simulink model "Control_v6_LQR_2020b"  (R2020b)
settings: Solver=FixedStepAuto  StartTime=0.0  StopTime=t_sim  FixedStep=TimeStep  RelTol=1e-3
values from neighbouring files (symbols this model uses):
  R = [ 1    0            0;         0    cos(alpha)  -sin(alpha);         0    sin(alpha)   cos(alpha)]    [main_SCA_v3.m]    (also in main_SCA_v3_alt.m; main_SCA_v4_LQR.m; main_SCA_v5.m)
  Use_IGRF = 0    [main_SCA.m]    (also in main_SCA_v3.m; main_SCA_v3_alt.m; main_SCA_v4_LQR.m; main_SCA_v5.m = 1)
undefined symbols (not defined in the file or in its folder): att, C, date, deg, DiscIntNeverNeededParam, IonSataero, Isat_inverse, km, orbit, Q, rad, s, sat
libraries: vrlib x23, aerolibutil x16, dspmathops x15, aerolibconvert2 x14, sharedtransform x13, simulink x4, simulink_extras x2, aerolibatmos2 x1, DipoleModel x1, aerolibobsolete x1, sharedutil x1, aerolibcelestial x1
(part 2 of 4)

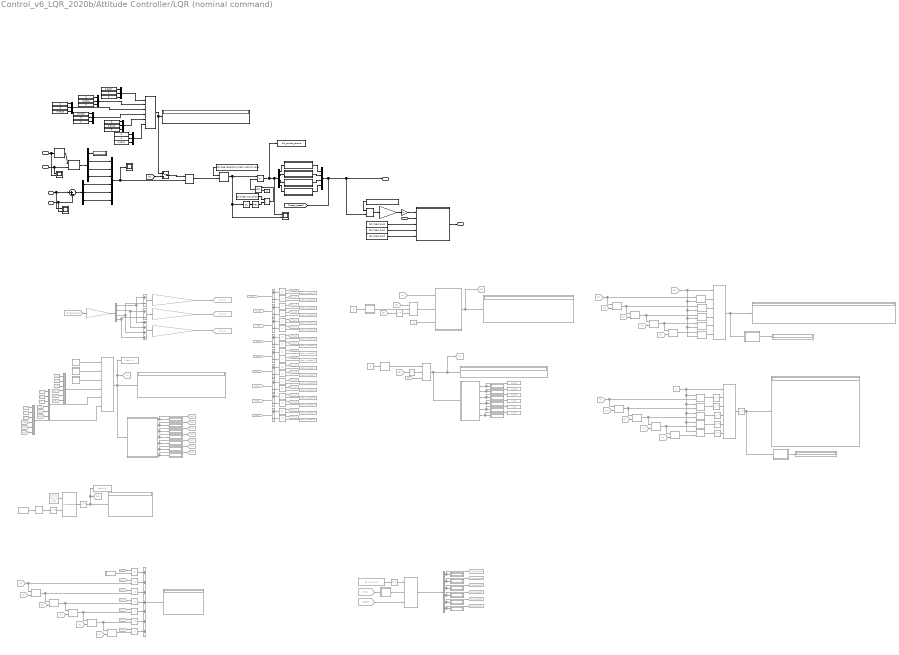
== system Control_v6_LQR_2020b/Attitude Controller/LQR (nominal command) ==
  note: Observability matrix [Ob]
  note: Feedback gain obtained by solving the algebraic Riccati equation
  note: Algebraic Riccati equation solver
  note: Feedback gain matrix K from the Ackerman's formula
  note: The dynamic of the corrected system is contained is the polynomial P_BF(A)
  note: State-space A matrix and its characteristic polynomial coefficients
  note: State-space B matrix
  note: Governability or Controllability matrix Gv
  note: on projete T dans
      | le plan perpendiculaire à B ?
      | Pas obligatoire (cf définition des blocs)
  note: See https://en.wikipedia.org/wiki/Rotation_formalisms_in_three_dimensions Quaternion <=> Angular velocity
      |
      | See http://www.diva-portal.org/smash/get/diva2:1020537/FULLTEXT02.pdf for 6DOF equations (3.13 p15)
      |
      | With ω = rotation vector (Omega_body) we have :
      |
      | $\frac{dω}{dt} = \hat{I}^{-1} [−ω(t) × (I_{Total}ω(t) + h_{RW}) + T_{dist}(t) − \frac{dh_{RW}}{dt} ̇ ]$
      | and with $\hat{I}=I_{Total}-L*I_{RW}*L^T$
  note: Computing the coefficient of the matrix A
  B_IGRF_Body : Inport
  q_ref : Inport  Port=2
  Q_ECI : Inport  Port=3
  W_Body : Inport  Port=4
  W_ref : Inport  Port=5
  Abs2 : Abs
  Algebraic Riccati equation solver : MATLAB Function  Commented=on  TreatAsAtomicUnit=on
  Command Magnetic moments computation : Subsystem
  Constant : Constant  Value=sat.wheel.repartition_matrix_4RW
  Constant1 : Constant  Commented=on  Value=[0 0 0 0 0 1]
  Constant10 : Constant  Commented=on  Value=Isat_inverse(7)
  Constant11 : Constant  Commented=on  Value=Isat_inverse(8)
  Constant12 : Constant  Value=sat.mag_t.axe1
  Constant13 : Constant  Value=sat.mag_t.axe2
  Constant14 : Constant  Value=sat.mag_t.axe3
  Constant15 : Constant  Commented=on  Value=Isat_inverse(9)
  Constant16 : Constant  Commented=on  Value=Isat_inverse(7)
  Constant17 : Constant  Commented=on  Value=Isat_inverse(8)
  Constant18 : Constant  Commented=on  Value=Isat_inverse(9)
  Constant19 : Constant  Commented=on  Value=Isat_inverse(1)
  Constant2 : Constant  Commented=on  Value=Isat_inverse(1)
  Constant20 : Constant  Commented=on  Value=Isat_inverse(2)
  Constant21 : Constant  Commented=on  Value=Isat_inverse(3)
  Constant22 : Constant  Commented=on  Value=Isat_inverse(4)
  Constant23 : Constant  Commented=on  Value=Isat_inverse(5)
  Constant24 : Constant  Commented=on  Value=Isat_inverse(6)
  Constant25 : Constant  Commented=on  Value=1/2
  Constant{26..28,30..32} (6 alike) : Constant  Commented=on  Value=0
  Constant29 : Constant  Commented=on  Value=1/2
  Constant3 : Constant  Commented=on  Value=Isat_inverse(2)
  Constant33 : Constant  Commented=on  Value=1/2
  Constant34 : Constant  Commented=on  Value=[0 0 0; 0 0 0; 0 0 0]
  Constant35 : Constant  Commented=on  Value=sat.inertia
  Constant36 : Constant  Commented=on  Value=R
  Constant37 : Constant  Value=sat.wheel.max_torque
  Constant38 : Constant
  Constant39 : Constant  Commented=on  Value=Q
  Constant4 : Constant  Commented=on  Value=Isat_inverse(3)
  Constant{6,40,42..43,46..48,51,53..56} (12 alike) : Constant  Value=0
  Constant41 : Constant  Commented=on  Value=R
  Constant44 : Constant  Value=0.0151
  Constant45 : Constant  Value=0.0017
  Constant49 : Constant  Value=0.0122
  Constant5 : Constant  Commented=on  Value=Isat_inverse(4)
  Constant50 : Constant  Commented=on  Value=C
  Constant52 : Constant  Value=0.0103
  Constant57 : Constant  Value=0.0016
  Constant7 : Constant  Value=0.0016
  Constant8 : Constant  Commented=on  Value=Isat_inverse(5)
  Constant9 : Constant  Commented=on  Value=Isat_inverse(6)
  Demux : Demux
  Demux4 : Demux  Commented=on
  Demux6 : Demux  Commented=on  Outputs=6
  Demux7 : Demux
  Demux8 : Demux  Outputs=3
  Display : Display
  Display{1..19,21..22,26,31..36} (28 alike) : Display  Commented=on
  Display20 : Display
  Divide1 : Product  Inputs=*/
  From : From  Commented=on  GotoTag=A44
  From100 : From  Commented=on  GotoTag=a6
  From{76..80,82..87,103,106,109..112} (17 alike) : From  Commented=on
  From{70,104..105,108} (4 alike) : From  Commented=on  GotoTag=B
  From107 : From  Commented=on  GotoTag=P
  From13 : From  Commented=on  GotoTag=Wheel_speed
  From31 : From  Commented=on  GotoTag=A54
  From32 : From  Commented=on  GotoTag=A64
  From33 : From  Commented=on  GotoTag=A45
  From{34,40,43,46,50,53} (6 alike) : From  Commented=on  GotoTag=hw_x
  From{35,41,44,47,56..57} (6 alike) : From  Commented=on  GotoTag=hw_z
  From{36,42,45,51..52,54} (6 alike) : From  Commented=on  GotoTag=hw_y
  From64 : From  Commented=on  GotoTag=A55
  From65 : From  Commented=on  GotoTag=A65
  From66 : From  Commented=on  GotoTag=A46
  From67 : From  Commented=on  GotoTag=A56
  From68 : From  Commented=on  GotoTag=A66
  From88 : From  Commented=on  GotoTag=Gv
  From89 : From  Commented=on  GotoTag=P_BF
  From94 : From  Commented=on  GotoTag=a0
  From95 : From  Commented=on  GotoTag=a1
  From96 : From  Commented=on  GotoTag=a2
  From97 : From  Commented=on  GotoTag=a3
  From98 : From  Commented=on  GotoTag=a4
  From99 : From  Commented=on  GotoTag=a5
  Gain1 : Gain
  Gain2 : Gain  Commented=on  Gain=sat.wheel.inertia
  Goto1 : Goto  Commented=on  GotoTag=A44
  Goto10 : Goto  Commented=on  GotoTag=A54
  Goto11 : Goto  Commented=on  GotoTag=hw_x
  Goto12 : Goto  Commented=on  GotoTag=hw_y
  Goto13 : Goto  Commented=on  GotoTag=hw_z
  Goto14 : Goto  Commented=on  GotoTag=A55
  Goto15 : Goto  Commented=on  GotoTag=A56
  Goto16 : Goto  Commented=on  GotoTag=A64
  Goto17 : Goto  Commented=on  GotoTag=A65
  Goto18 : Goto  Commented=on  GotoTag=A66
  Goto19 : Goto  Commented=on
  Goto2 : Goto  Commented=on  GotoTag=K
  Goto20 : Goto  Commented=on  GotoTag=B
  Goto21 : Goto  Commented=on  GotoTag=a5
  Goto23 : Goto  Commented=on  GotoTag=a4
  Goto24 : Goto  Commented=on  GotoTag=a3
  Goto25 : Goto  Commented=on  GotoTag=a2
  Goto26 : Goto  Commented=on  GotoTag=a1
  Goto27 : Goto  Commented=on  GotoTag=a0
  Goto28 : Goto  Commented=on  GotoTag=a6
  Goto30 : Goto  Commented=on  GotoTag=P
  Goto31 : Goto  Commented=on  GotoTag=k_que2_ack
  Goto32 : Goto  Commented=on  GotoTag=k_que3_ack
  Goto34 : Goto  Commented=on  GotoTag=k_wb1_ack
  Goto35 : Goto  Commented=on  GotoTag=k_wb2_ack
  Goto36 : Goto  Commented=on  GotoTag=k_wb3_ack
  Goto37 : Goto  Commented=on  GotoTag=k_que1_ack
  Goto8 : Goto  Commented=on  GotoTag=A45
  Goto9 : Goto  Commented=on  GotoTag=A46
  IdentityMatrix [6x6] : Subsystem  Description=Replaced Block  Commented=on  mask(Replaced Block){}
      mask help: This block has been replaced with an empty subsystem because it used functionality that is unavailable in Simulink R2020b.
      mask Display: fprintf('Replaced: %s\n','IdentityMatrix')
  Inverse nxn matrix : MATLAB Function  Commented=on  TreatAsAtomicUnit=on
  Inverse nxn matrix1 : MATLAB Function  Commented=on  TreatAsAtomicUnit=on
  Inverse nxn matrix2 : MATLAB Function  Commented=on  TreatAsAtomicUnit=on
  Invert 3x3 Matrix : aerolibutil/Invert  3x3 Matrix  Commented=on
  Is the system controllable? : MATLAB Function  Commented=on  TreatAsAtomicUnit=on
  Is the system observable? : MATLAB Function  Commented=on  TreatAsAtomicUnit=on
  Manual Switch : ManualSwitch
  Matrix Concatenate : Concatenate  Commented=on  NumInputs=6  Mode=Multidimensional array  ConcatenateDimension=2
  Matrix Concatenate1 : Concatenate  Commented=on  Mode=Multidimensional array  ConcatenateDimension=2
  Matrix Concatenate2 : Concatenate  Commented=on  NumInputs=6  Mode=Multidimensional array  ConcatenateDimension=2
  Matrix Concatenate3 : Concatenate  Commented=on  NumInputs=6  Mode=Multidimensional array  ConcatenateDimension=2
  Matrix Concatenate4 : Concatenate  NumInputs=6  Mode=Multidimensional array  ConcatenateDimension=2
  Matrix Multiply{,1..13,17..25} (23 alike) : Product  Commented=on  Multiplication=Matrix(*)
  Matrix Multiply14 : Product  Commented=on  Inputs=3  Multiplication=Matrix(*)
  Matrix Multiply15 : Product  Commented=on  Inputs=3  Multiplication=Matrix(*)
  Matrix Multiply16 : Product  Commented=on  Inputs=3  Multiplication=Matrix(*)
  MatrixMultiply1 : Product  Multiplication=Matrix(*)
  MatrixMultiply2 : Product  Multiplication=Matrix(*)
  MatrixMultiply3 : Product  Multiplication=Matrix(*)
  Max of Elements2 : MinMax  Function=max
  Min1 : MinMax  Inputs=2
  Mux : Mux
  Mux5 : Mux  Inputs=6
  Product{2..12,31..37,54..60} (25 alike) : Product  Commented=on
  Product13 : Product
  Quaternion Inverse : aerolibutil/Quaternion Inverse
  Quaternion Multiplication : aerolibutil/Quaternion Multiplication
  RW1 : Subsystem
  RW2 : Subsystem
  RW3 : Subsystem
  "RW4 " : Subsystem
  Repartition RWA1 : Constant  Value=sat.wheel.repartition_metrix_4RW_inverse
  Scope : Scope
  Scope1 : Scope  NumInputPorts=2
  Scope2 : Scope  NumInputPorts=2
  Scope3 : Scope  NumInputPorts=2
  Sum{7,11,13..21} (11 alike) : Sum  Commented=on  Inputs=+-
  Sum12 : Sum  Commented=on  Inputs=++++
  Sum25 : Sum  Inputs=|+-
  Sum26 : Sum  Commented=on  Inputs=+++++++
  To Workspace11 : ToWorkspace  VariableName=RW_control_torque  SaveFormat=Timeseries  SampleTime=-1
  To Workspace2 : ToWorkspace  Commented=on  VariableName=Matrix_A  SaveFormat=Timeseries  SampleTime=-1
  To Workspace3 : ToWorkspace  Commented=on  VariableName=Matrix_B  SaveFormat=Timeseries  SampleTime=-1
  To Workspace4 : ToWorkspace  Commented=on  VariableName=k_qe1  SaveFormat=Timeseries  SampleTime=-1
  To Workspace5 : ToWorkspace  Commented=on  VariableName=k_qe2  SaveFormat=Timeseries  SampleTime=-1
  To Workspace6 : ToWorkspace  Commented=on  VariableName=k_qe3  SaveFormat=Timeseries  SampleTime=-1
  To Workspace7 : ToWorkspace  Commented=on  VariableName=k_w1  SaveFormat=Timeseries  SampleTime=-1
  To Workspace8 : ToWorkspace  Commented=on  VariableName=k_w2  SaveFormat=Timeseries  SampleTime=-1
  To Workspace9 : ToWorkspace  Commented=on  VariableName=k_w3  SaveFormat=Timeseries  SampleTime=-1
  Transpose{,1..10} (11 alike) : Math  Commented=on  Operator=transpose  SaturateOnIntegerOverflow=on
  Vector Concatenate : Concatenate  Commented=on  NumInputs=6
  Vector Concatenate1 : Concatenate  Commented=on  NumInputs=6
  Vector Concatenate2 : Concatenate  Commented=on  NumInputs=6
  Vector Concatenate{3..8} (6 alike) : Concatenate  NumInputs=3
  "[0 ... 0]^T" : Subsystem  Commented=on
  "[0 .... 0]^T" : Subsystem  Commented=on
  "[0 0 0 0 0 0]^T " : Subsystem  Commented=on
  cos(beta) : Gain  Commented=on  Gain=sat.wheel.repartition_matrix_4RW(1)
  cos(beta)1 : Gain  Commented=on  Gain=sat.wheel.repartition_matrix_4RW(1)
  kp_mag : Gain  Gain=sat.PID.kpmag
  returns the feedback gain that are used : MATLAB Function  Commented=on  TreatAsAtomicUnit=on
  returns the n+1 = 7 coefficients of the characteristics polynomial of the matrix A : MATLAB Function  Commented=on  TreatAsAtomicUnit=on
  sin(beta) : Gain  Commented=on  Gain=sat.wheel.repartition_matrix_4RW(9)
  RW Command : Outport  VectorParamsAs1DForOutWhenUnconnected=off
  Mag Command : Outport  Port=2  VectorParamsAs1DForOutWhenUnconnected=off
  wires:
  Command Magnetic moments computation/1(Mag vector command) -> Mag Command/1
  Constant14/1 -> Command Magnetic moments computation/5(h3 (vect))
  Constant12/1 -> Command Magnetic moments computation/3(h1 (vect))
  Constant/1 -> MatrixMultiply1/1
  Demux/4 -> "RW4 "/1(Mc (scalar))
  Constant13/1 -> Command Magnetic moments computation/4(h2 (vect))
  Demux/3 -> RW3/1(Mc (scalar))
  RW3/1(Omega_C (scalar)) -> Mux/3
  RW2/1(Omega_C (scalar)) -> Mux/2
  Demux/2 -> RW2/1(Mc (scalar))
  Demux/1 -> RW1/1(Mc (scalar))
  Gain1/1 -> Command Magnetic moments computation/1(Command (vect))
  B_IGRF_Body/1 -> Command Magnetic moments computation/2(B_IGRF_body (vect))
  "RW4 "/1(Omega_C (scalar)) -> Mux/4
  kp_mag/1 -> Gain1/1
  MatrixMultiply1/1 -> kp_mag/1
  RW1/1(Omega_C (scalar)) -> Mux/1
  Mux/1 -> [Wheel_speed], MatrixMultiply1/2, RW Command/1  "rad/s"
  Gain2/1 -> Demux4/1
  Demux4/2 -> Sum12/2, Sum7/1
  Demux4/1 -> Sum12/1, Sum11/1  "Iw1*omega_wheel1  (kg.m².s^-1"
  Demux4/3 -> Sum12/3, Sum11/2
  Demux4/4 -> Sum12/4, Sum7/2
  Sum7/1 -> cos(beta)1/1
  Sum11/1 -> cos(beta)/1
  Sum12/1 -> sin(beta)/1
  cos(beta)/1 -> Goto11/1  "hw_x  (kg.m².s^-1)"
  cos(beta)1/1 -> Goto12/1  "hw_y  (kg.m².s^-1)"
  sin(beta)/1 -> Goto13/1  "hw_z  (kg.m².s^-1)"
  Sum13/1 -> Goto1/1  "A44"
  Sum14/1 -> Goto8/1  "A45"
  Sum15/1 -> Goto9/1  "A46"
  Sum16/1 -> Goto10/1  "A54"
  Sum19/1 -> Goto14/1  "A55"
  Sum18/1 -> Goto15/1  "A56"
  Sum20/1 -> Goto16/1  "A64"
  Sum21/1 -> Goto17/1  "A65"
  Sum17/1 -> Goto18/1  "A66"
  Product3/1 -> Sum13/2
  Product2/1 -> Sum13/1
  Product5/1 -> Sum14/2
  Product4/1 -> Sum14/1
  Product7/1 -> Sum15/2
  Product6/1 -> Sum15/1
  Product9/1 -> Sum16/2
  Product8/1 -> Sum16/1
  Product11/1 -> Sum17/2
  Product10/1 -> Sum17/1
  Product31/1 -> Sum18/2
  Product12/1 -> Sum18/1
  Product33/1 -> Sum19/2
  Product32/1 -> Sum19/1
  Product35/1 -> Sum20/2
  Product34/1 -> Sum20/1
  Product37/1 -> Sum21/2
  Product36/1 -> Sum21/1
  From35/1 -> Product2/1
  From36/1 -> Product3/1
  Constant3/1 -> Product2/2
  Constant4/1 -> Product3/2
  From34/1 -> Product4/1
  Constant21/1 -> Product4/2
  From41/1 -> Product5/1
  Constant2/1 -> Product5/2
  From42/1 -> Product6/1
  From40/1 -> Product7/1
  Constant19/1 -> Product6/2
  Constant20/1 -> Product7/2
  Constant8/1 -> Product8/2
  Constant9/1 -> Product9/2
  Constant22/1 -> Product33/2
  Constant24/1 -> Product32/2
  From44/1 -> Product8/1
  From45/1 -> Product9/1
  From43/1 -> Product32/1
  From47/1 -> Product33/1
  Constant5/1 -> Product12/2
  Constant23/1 -> Product31/2
  From52/1 -> Product12/1
  From50/1 -> Product31/1
  Constant11/1 -> Product34/2
  Constant15/1 -> Product35/2
  Constant18/1 -> Product36/2
  Constant10/1 -> Product37/2
  Constant16/1 -> Product10/2
  Constant17/1 -> Product11/2
  From56/1 -> Product34/1
  From51/1 -> Product35/1
  From53/1 -> Product36/1
  From57/1 -> Product37/1
  From54/1 -> Product10/1
  From46/1 -> Product11/1
  q_ref/1 -> Scope3/1, Quaternion Multiplication/2
  "[0 ... 0]^T"/1(Out1) -> Matrix Concatenate/3  "Ai3 colum vector"
  "[0 0 0 0 0 0]^T "/1(Out1) -> Matrix Concatenate/1  "Ai1 colum vector"
  "[0 .... 0]^T"/1(Out1) -> Matrix Concatenate/2  "Ai2 colum vector"
  Matrix Concatenate/1 -> returns the n+1 = 7 coefficients of the characteristics polynomial of the matrix A/1(A), To Workspace2/1, Goto19/1, Display1/1  "State-space matrix [A]"
  From31/1 -> Vector Concatenate/5
  Constant26/1 -> Vector Concatenate/2
  Vector Concatenate/1 -> Matrix Concatenate/4  "Ai4 colum vector"
  From32/1 -> Vector Concatenate/6
  Constant25/1 -> Vector Concatenate/1
  Constant27/1 -> Vector Concatenate/3
  From/1 -> Vector Concatenate/4
  From33/1 -> Vector Concatenate1/4
  Vector Concatenate1/1 -> Matrix Concatenate/5  "Ai5 colum vector"
  Constant30/1 -> Vector Concatenate1/3
  Constant28/1 -> Vector Concatenate1/1
  From64/1 -> Vector Concatenate1/5
  Constant29/1 -> Vector Concatenate1/2
  From65/1 -> Vector Concatenate1/6
  From66/1 -> Vector Concatenate2/4
  Vector Concatenate2/1 -> Matrix Concatenate/6  "Ai6 colum vector"
  Constant33/1 -> Vector Concatenate2/3
  Constant31/1 -> Vector Concatenate2/1
  From67/1 -> Vector Concatenate2/5
  Constant32/1 -> Vector Concatenate2/2
  From68/1 -> Vector Concatenate2/6
  Constant34/1 -> Matrix Concatenate1/1
  Transpose2/1 -> Matrix Concatenate1/2
  Matrix Concatenate1/1 -> Transpose1/1
  Transpose1/1 -> To Workspace3/1, Goto20/1, Display4/1  "State-space matrix [B]"
  Constant35/1 -> Invert 3x3 Matrix/1
  Invert 3x3 Matrix/1 -> Transpose2/1  "Isat^-1"
  Matrix Multiply/1 -> Matrix Concatenate2/2  "[Gv]i2"
  Matrix Multiply1/1 -> Matrix Concatenate2/3  "[Gv]i3"
  Matrix Multiply2/1 -> Matrix Concatenate2/4  "[Gv]i4"
  Matrix Multiply3/1 -> Matrix Concatenate2/5  "[Gv]i5"
  Matrix Multiply4/1 -> Matrix Concatenate2/6  "[Gv]i6"
  From70/1 -> Matrix Multiply/2, Matrix Multiply1/2, Matrix Multiply2/2, Matrix Multiply3/2, Matrix Multiply4/2, Matrix Concatenate2/1  "[Gv]i1"
  From76/1 -> Matrix Multiply5/1, Matrix Multiply/1
  From77/1 -> Matrix Multiply5/2
  Matrix Multiply5/1 -> Matrix Multiply6/1, Matrix Multiply1/1  "A^2"
  From78/1 -> Matrix Multiply6/2
  From79/1 -> Matrix Multiply7/2
  Matrix Multiply6/1 -> Matrix Multiply7/1, Matrix Multiply2/1  "A^3"
  Matrix Multiply7/1 -> Matrix Multiply8/1, Matrix Multiply3/1  "A^4"
  From80/1 -> Matrix Multiply8/2
  Matrix Multiply8/1 -> Matrix Multiply4/1  "A^5"
  Matrix Concatenate2/1 -> Display3/1, Is the system controllable?/1(Gv)  "Controllability matrix [Gv]"
  returns the n+1 = 7 coefficients of the characteristics polynomial of the matrix A/1(a6) -> Goto28/1, Display2/1
  returns the n+1 = 7 coefficients of the characteristics polynomial of the matrix A/3(a4) -> Display6/1, Goto23/1
  returns the n+1 = 7 coefficients of the characteristics polynomial of the matrix A/4(a3) -> Display7/1, Goto24/1
  returns the n+1 = 7 coefficients of the characteristics polynomial of the matrix A/5(a2) -> Display8/1, Goto25/1
  returns the n+1 = 7 coefficients of the characteristics polynomial of the matrix A/6(a1) -> Goto26/1, Display9/1
  returns the n+1 = 7 coefficients of the characteristics polynomial of the matrix A/7(a0) -> Display10/1, Goto27/1
  returns the n+1 = 7 coefficients of the characteristics polynomial of the matrix A/2(a5) -> Goto21/1, Display5/1
  Is the system controllable?/1(y) -> Display11/1
  Matrix Multiply11/1 -> Product58/2, Matrix Multiply12/1  "A^4"
  Matrix Multiply9/1 -> Product56/2, Matrix Multiply10/1  "A^2"
  Matrix Multiply10/1 -> Product57/2, Matrix Multiply11/1  "A^3"
  From83/1 -> Matrix Multiply9/2
  From86/1 -> Matrix Multiply12/2
  From85/1 -> Matrix Multiply11/2
  From84/1 -> Matrix Multiply10/2
  From82/1 -> Product55/2, Matrix Multiply9/1
  From94/1 -> Product54/1
  IdentityMatrix [6x6]/1(Out1) -> Product54/2
  Product54/1 -> Sum26/1
  From95/1 -> Product55/1
  Product55/1 -> Sum26/2
  From96/1 -> Product56/1
  Product56/1 -> Sum26/3
  From97/1 -> Product57/1
  Product57/1 -> Sum26/4
  From98/1 -> Product58/1
  Product58/1 -> Sum26/5
  From99/1 -> Product59/1
  Product59/1 -> Sum26/6
  From100/1 -> Product60/1
  Product60/1 -> Sum26/7
  Sum26/1 -> Display12/1  "[P_BF(A)]"
  Matrix Multiply12/1 -> Matrix Multiply13/1, Product59/2  "A^5"
  From87/1 -> Matrix Multiply13/2
  Matrix Multiply13/1 -> Product60/2  "A^6"
  Matrix Multiply14/1 -> Demux6/1  "Feedback gain matrix [K]"
  Constant1/1 -> Transpose3/1
  Transpose3/1 -> Matrix Multiply14/1
  From89/1 -> Matrix Multiply14/3
  From88/1 -> Inverse nxn matrix/1(u)
  Inverse nxn matrix/1(y) -> Matrix Multiply14/2  "[Gv]^-1"
  Demux6/1 -> Goto37/1, Display14/1
  Demux6/4 -> Goto34/1, Display18/1
  Demux6/6 -> Display13/1, Goto36/1
  Demux6/3 -> Display16/1, Goto32/1
  Demux6/5 -> Goto35/1, Display19/1
  Demux6/2 -> Goto31/1, Display15/1
  From103/1 -> Algebraic Riccati equation solver/1(A)
  Matrix Multiply15/1 -> Algebraic Riccati equation solver/2(G)
  From104/1 -> Matrix Multiply15/1
  From105/1 -> Transpose/1
  Transpose/1 -> Matrix Multiply15/3
  Inverse nxn matrix1/1(y) -> Matrix Multiply15/2  "[R]^-1"
  Algebraic Riccati equation solver/1(P) -> Goto30/1, Display17/1  "solution of the Riccati equation"
  Constant39/1 -> Algebraic Riccati equation solver/3(Q)
  Transpose4/1 -> Matrix Multiply16/2
  Constant41/1 -> Inverse nxn matrix2/1(u)
  Inverse nxn matrix2/1(y) -> Matrix Multiply16/1  "[R]^-1"
  From108/1 -> Transpose4/1
  From107/1 -> Matrix Multiply16/3
  Matrix Multiply16/1 -> returns the feedback gain that are used/1(K), Goto2/1, Display26/1  "Feedbak gain matrix [K]"
  Constant36/1 -> Inverse nxn matrix1/1(u)
  Quaternion Inverse/1 -> Quaternion Multiplication/1
  Q_ECI/1 -> Scope3/2, Quaternion Inverse/1
  W_ref/1 -> Scope2/2, Sum25/2
  W_Body/1 -> Sum25/1, Scope2/1
  Quaternion Multiplication/1 -> Demux7/1  "Qr"
  Matrix Concatenate3/1 -> Transpose5/1
  Transpose6/1 -> Matrix Concatenate3/2
  Constant50/1 -> Matrix Concatenate3/1, Matrix Multiply17/1, Matrix Multiply19/1, Matrix Multiply20/1, Matrix Multiply21/1, Matrix Multiply18/1
  From112/1 -> Matrix Multiply25/2
  Matrix Multiply25/1 -> Matrix Multiply21/2  "A^5"
  From109/1 -> Matrix Multiply22/2
  Matrix Multiply23/1 -> Matrix Multiply24/1, Matrix Multiply19/2  "A^3"
  Matrix Multiply24/1 -> Matrix Multiply20/2, Matrix Multiply25/1  "A^4"
  From111/1 -> Matrix Multiply24/2
  Matrix Multiply22/1 -> Matrix Multiply23/1, Matrix Multiply18/2  "A^2"
  From106/1 -> Matrix Multiply17/2, Matrix Multiply22/1
  From110/1 -> Matrix Multiply23/2
  Demux8/3 -> Mux5/6  "W_error_3"
  Demux8/1 -> Mux5/4  "W_error_1"
  Demux7/2 -> Mux5/1  "Q_error_1"
  Demux8/2 -> Mux5/5  "W_error_2"
  Demux7/4 -> Mux5/3  "Q_error_3"
  Demux7/3 -> Mux5/2  "Q_error_2"
  Sum25/1 -> Demux8/1
  Demux7/1 -> Display20/1
  Mux5/1 -> MatrixMultiply2/2, Scope/1  "x_error(t)"
  Transpose7/1 -> Matrix Concatenate3/3
  Transpose9/1 -> Matrix Concatenate3/5
  Transpose8/1 -> Matrix Concatenate3/4
  Transpose10/1 -> Matrix Concatenate3/6
  Matrix Multiply21/1 -> Transpose10/1
  Matrix Multiply20/1 -> Transpose9/1
  Matrix Multiply19/1 -> Transpose8/1
  Matrix Multiply18/1 -> Transpose7/1
  Matrix Multiply17/1 -> Transpose6/1
  Is the system observable?/1(y) -> Display21/1
  Transpose5/1 -> Is the system observable?/1(Gv), Display22/1  "Observability matrix [Ob]"
  returns the feedback gain that are used/1(k_qe1) -> To Workspace4/1, Display31/1  "K11"
  returns the feedback gain that are used/2(k_qe2) -> To Workspace5/1, Display32/1  "K22"
  returns the feedback gain that are used/6(k_w3) -> To Workspace9/1, Display36/1  "K36"
  returns the feedback gain that are used/5(k_w2) -> To Workspace8/1, Display35/1  "K25"
  returns the feedback gain that are used/4(k_w1) -> To Workspace7/1, Display34/1  "K14"
  returns the feedback gain that are used/3(k_qe3) -> To Workspace6/1, Display33/1  "K33"
  From13/1 -> Gain2/1
  Matrix Concatenate4/1 -> Manual Switch/1, Display/1
  Repartition RWA1/1 -> MatrixMultiply3/1
  MatrixMultiply2/1 -> MatrixMultiply3/2  "(kg.m².s^-2)"
  Abs2/1 -> Max of Elements2/1
  Constant37/1 -> Divide1/1
  Min1/1 -> Product13/2
  Divide1/1 -> Min1/1
  Constant38/1 -> Min1/2
  Max of Elements2/1 -> Divide1/2
  Product13/1 -> To Workspace11/1, Scope1/1, Demux/1  "T limit"
  MatrixMultiply3/1 -> Scope1/2, Abs2/1, Product13/1
  [K] -> Manual Switch/2
  Manual Switch/1 -> MatrixMultiply2/1
  Constant47/1 -> Vector Concatenate5/3
  Vector Concatenate5/1 -> Matrix Concatenate4/1  "Ki1 colum vector"
  Constant46/1 -> Vector Concatenate5/2
  Constant45/1 -> Vector Concatenate5/1
  Constant7/1 -> Vector Concatenate3/2
  Constant40/1 -> Vector Concatenate3/3
  Constant6/1 -> Vector Concatenate3/1
  Vector Concatenate3/1 -> Matrix Concatenate4/2  "Ki2 colum vector"
  Constant43/1 -> Vector Concatenate4/2
  Constant44/1 -> Vector Concatenate4/3
  Constant42/1 -> Vector Concatenate4/1
  Vector Concatenate4/1 -> Matrix Concatenate4/6  "Ki6 colum vector"
  Constant49/1 -> Vector Concatenate6/2
  Constant51/1 -> Vector Concatenate6/3
  Constant48/1 -> Vector Concatenate6/1
  Vector Concatenate6/1 -> Matrix Concatenate4/5  "Ki5 colum vector"
  Constant53/1 -> Vector Concatenate7/2
  Constant54/1 -> Vector Concatenate7/3
  Constant52/1 -> Vector Concatenate7/1
  Vector Concatenate7/1 -> Matrix Concatenate4/4  "Ki4 colum vector"
  Constant56/1 -> Vector Concatenate8/2
  Constant57/1 -> Vector Concatenate8/3
  Constant55/1 -> Vector Concatenate8/1
  Vector Concatenate8/1 -> Matrix Concatenate4/3  "Ki3 colum vector"

== system Control_v6_LQR_2020b/Attitude Controller/Magnetorquer Magnetic Momend Command ==
  " command (normal)" : Inport
  Command (B-dot) : Inport  Port=2
  B_dot mode (0/1) : Inport  Port=3
  If1 : If
  Merge : Merge
  Switch Case Action Subsystem3 : Subsystem  TreatAsAtomicUnit=on
  Switch Case Action Subsystem4 : Subsystem  TreatAsAtomicUnit=on
  output command : Outport  VectorParamsAs1DForOutWhenUnconnected=off
  wires:
  If1/2 -> Switch Case Action Subsystem4/Action
  If1/1 -> Switch Case Action Subsystem3/Action
  B_dot mode (0/1)/1 -> If1/1
  Command (B-dot)/1 -> Switch Case Action Subsystem3/1(In1)
  Switch Case Action Subsystem3/1(Out1) -> Merge/1
  Switch Case Action Subsystem4/1(Out1) -> Merge/2
  " command (normal)"/1 -> Switch Case Action Subsystem4/1(In1)
  Merge/1 -> output command/1

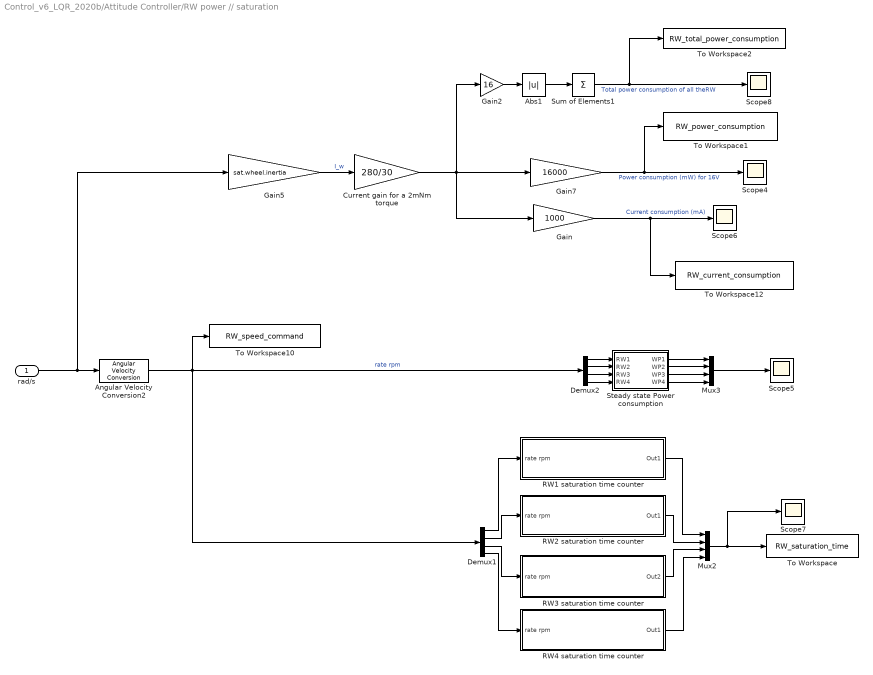
== system Control_v6_LQR_2020b/Attitude Controller/RW power // saturation ==
  rad/s : Inport
  Abs1 : Abs
  Angular Velocity Conversion2 : aerolibconvert2/Angular Velocity Conversion  IU=rad/s  OU=rpm
  Current gain for a 2mNm torque : Gain  Gain=280/30
  Demux1 : Demux
  Demux2 : Demux
  Gain : Gain  Gain=1000
  Gain2 : Gain  Gain=16
  Gain5 : Gain  Gain=sat.wheel.inertia
  Gain7 : Gain  Gain=16000
  Mux2 : Mux
  Mux3 : Mux
  RW1 saturation time counter : Subsystem
  RW2 saturation time counter : Subsystem
  RW3 saturation time counter : Subsystem
  RW4 saturation time counter : Subsystem
  Scope{4..8} (5 alike) : Scope
  Steady state Power consumption : MATLAB Function  TreatAsAtomicUnit=on
  Sum of Elements1 : Sum  Inputs=+
  To Workspace : ToWorkspace  VariableName=RW_saturation_time  SaveFormat=Timeseries  SampleTime=-1
  To Workspace1 : ToWorkspace  VariableName=RW_power_consumption  SaveFormat=Timeseries  SampleTime=-1
  To Workspace10 : ToWorkspace  VariableName=RW_speed_command  SaveFormat=Timeseries  SampleTime=-1
  To Workspace12 : ToWorkspace  VariableName=RW_current_consumption  SaveFormat=Timeseries  SampleTime=-1
  To Workspace2 : ToWorkspace  VariableName=RW_total_power_consumption  SaveFormat=Timeseries  SampleTime=-1
  wires:
  Demux1/3 -> RW3 saturation time counter/1(rate rpm)
  RW2 saturation time counter/1(Out1) -> Mux2/2
  Abs1/1 -> Sum of Elements1/1
  Gain7/1 -> To Workspace1/1, Scope4/1  "Power consumption (mW) for 16V"
  Demux1/4 -> RW4 saturation time counter/1(rate rpm)
  Demux2/2 -> Steady state Power consumption/2(RW2)
  Mux2/1 -> Scope7/1, To Workspace/1
  Demux1/1 -> RW1 saturation time counter/1(rate rpm)
  Mux3/1 -> Scope5/1
  Sum of Elements1/1 -> To Workspace2/1, Scope8/1  "Total power consumption of all theRW"
  Demux1/2 -> RW2 saturation time counter/1(rate rpm)
  RW3 saturation time counter/1(Out2) -> Mux2/3
  rad/s/1 -> Gain5/1, Angular Velocity Conversion2/1
  Gain/1 -> To Workspace12/1, Scope6/1  "Current consumption (mA)"
  RW4 saturation time counter/1(Out1) -> Mux2/4
  Demux2/3 -> Steady state Power consumption/3(RW3)
  Gain2/1 -> Abs1/1
  Gain5/1 -> Current gain for a 2mNm torque/1  "I_w"
  Demux2/4 -> Steady state Power consumption/4(RW4)
  RW1 saturation time counter/1(Out1) -> Mux2/1
  Angular Velocity Conversion2/1 -> Demux1/1, Demux2/1, To Workspace10/1  "rate rpm"
  Current gain for a 2mNm torque/1 -> Gain/1, Gain2/1, Gain7/1
  Steady state Power consumption/1(WP1) -> Mux3/1
  Steady state Power consumption/2(WP2) -> Mux3/2
  Steady state Power consumption/3(WP3) -> Mux3/3
  Demux2/1 -> Steady state Power consumption/1(RW1)
  Steady state Power consumption/4(WP4) -> Mux3/4

== system Control_v6_LQR_2020b/Attitude Controller/Reaction Wheels Speed Command ==
  " command (normal)" : Inport
  Command (B-dot) : Inport  Port=2
  B_dot mode (0/1) : Inport  Port=3
  If1 : If
  Merge : Merge
  Switch Case Action Subsystem3 : Subsystem  TreatAsAtomicUnit=on
  Switch Case Action Subsystem4 : Subsystem  TreatAsAtomicUnit=on
  output command : Outport  VectorParamsAs1DForOutWhenUnconnected=off
  wires:
  If1/2 -> Switch Case Action Subsystem4/Action
  If1/1 -> Switch Case Action Subsystem3/Action
  B_dot mode (0/1)/1 -> If1/1
  Command (B-dot)/1 -> Switch Case Action Subsystem3/1(In1)
  Merge/1 -> output command/1
  Switch Case Action Subsystem3/1(Out1) -> Merge/1
  Switch Case Action Subsystem4/1(Out1) -> Merge/2
  " command (normal)"/1 -> Switch Case Action Subsystem4/1(In1)

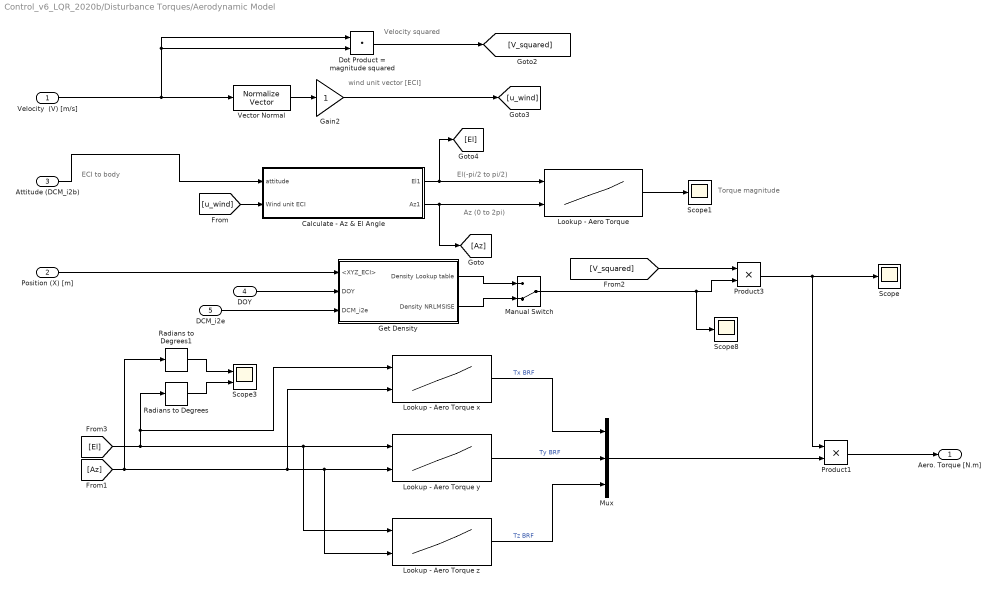
== system Control_v6_LQR_2020b/Disturbance Torques/Aerodynamic Model ==
  note: Az (0 to 2pi)
  note: wind unit vector [ECI]
  note: Torque magnitude
  note: ECI to body
  note: Velocity squared
  note: El(-pi/2 to pi/2)
  Velocity  (V) [m/s] : Inport
  Position (X) [m] : Inport  Port=2
  Attitude (DCM_i2b) : Inport  Port=3
  DOY : Inport  Port=4
  DCM_i2e : Inport  Port=5
  Calculate - Az & El Angle : Subsystem
  Dot Product = magnitude squared : DotProduct  InputSameDT=on  OutDataTypeStr=Inherit: Inherit via internal rule
  Gain2 : Gain
  Get Density : Subsystem
  Lookup - Aero Torque : Lookup2D  RowIndex=IonSataero.Az  ColumnIndex=IonSataero.El  Table=IonSataero.T
  Lookup - Aero Torque x : Lookup2D  RowIndex=IonSataero.Az  ColumnIndex=IonSataero.El  Table=IonSataero.Tx
  Lookup - Aero Torque y : Lookup2D  RowIndex=IonSataero.Az  ColumnIndex=IonSataero.El  Table=IonSataero.Ty
  Lookup - Aero Torque z : Lookup2D  RowIndex=IonSataero.Az  ColumnIndex=IonSataero.El  Table=IonSataero.Tz
  Manual Switch : ManualSwitch  CurrentSetting=0
  Mux : Mux  Inputs=3
  Product1 : Product  RndMeth=Zero
  Product3 : Product  RndMeth=Zero
  Radians to Degrees : simulink_extras/Transformations/Radians to Degrees
  Radians to Degrees1 : simulink_extras/Transformations/Radians to Degrees
  Scope : Scope
  Scope1 : Scope
  Scope3 : Scope  NumInputPorts=2
  Scope8 : Scope
  Vector Normal : vrlib/Utilities/Normalize Vector  maxzero=0
  Aero. Torque [N.m] : Outport
  wires:
  Dot Product = magnitude squared/1 -> [V_squared]
  Vector Normal/1 -> Gain2/1
  Gain2/1 -> [u_wind]
  Lookup - Aero Torque/1 -> Scope1/1
  Attitude (DCM_i2b)/1 -> Calculate - Az & El Angle/1(attitude)
  [V_squared] -> Product3/1
  Velocity  (V) [m/s]/1 -> Dot Product = magnitude squared/2, Dot Product = magnitude squared/1, Vector Normal/1
  Radians to Degrees1/1 -> Scope3/1
  Radians to Degrees/1 -> Scope3/2
  [u_wind] -> Calculate - Az & El Angle/2(Wind unit ECI)
  Calculate - Az & El Angle/2(Az1) -> [Az], Lookup - Aero Torque/2
  Calculate - Az & El Angle/1(El1) -> [El], Lookup - Aero Torque/1
  [El] -> Lookup - Aero Torque z/1, Lookup - Aero Torque y/1, Lookup - Aero Torque x/1, Radians to Degrees/1
  [Az] -> Radians to Degrees1/1, Lookup - Aero Torque z/2, Lookup - Aero Torque y/2, Lookup - Aero Torque x/2
  Lookup - Aero Torque y/1 -> Mux/2  "Ty BRF"
  Lookup - Aero Torque x/1 -> Mux/1  "Tx BRF"
  Lookup - Aero Torque z/1 -> Mux/3  "Tz BRF"
  Mux/1 -> Product1/2
  Product3/1 -> Product1/1, Scope/1
  Product1/1 -> Aero. Torque [N.m]/1
  Manual Switch/1 -> Scope8/1, Product3/2
  Position (X) [m]/1 -> Get Density/1(<XYZ_ECI>)
  DOY/1 -> Get Density/2(DOY)
  DCM_i2e/1 -> Get Density/3("DCM_i2e ")
  Get Density/2(Density NRLMSISE) -> Manual Switch/2
  Get Density/1(Density Lookup table) -> Manual Switch/1

== system Control_v6_LQR_2020b/Disturbance Torques/Gravity Gradient Model ==
  note: \tau_{gg}= 3\mu/r^{3} (u_{nadir}\times J* u_{nadir})
  note: (3*mu/Rs^4*) * Rs = (3*mu/Rs^3) * rs
  note: Nadir [body]
  note: position of satellite [ECI]
  note: Nadir unit vector
      | [body]
  note: Anti-nadir [body]
  note: r^4
  "Position (X) [m] " : Inport
  Attitude (DCMi2b) : Inport  Port=2
  3 * mu : Constant  Value=3*3.9860044188e14
  Cross Product : vrlib/Utilities/Cross Product
  Divide : Product  Inputs=*/
  Dot Product = magnitude squared : DotProduct  InputSameDT=on  OutDataTypeStr=Inherit: Inherit via internal rule
  Gain : Gain  Gain=-1
  Gain1 : Gain  Gain=-1
  J : Constant  Value=sat.inertia
  Math Function : Math  Operator=square  SignedPower=on  SaturateOnIntegerOverflow=on
  Product (not cross) : Product  RndMeth=Zero
  Vector Normal : vrlib/Utilities/Normalize Vector  maxzero=0
  product 1 : Product  Multiplication=Matrix(*)  RndMeth=Zero
  product 2 : Product  Multiplication=Matrix(*)  RndMeth=Zero
  Gravity Gradient [N.m] : Outport
  wires:
  Product (not cross)/1 -> Cross Product/1
  Divide/1 -> Product (not cross)/2
  3 * mu/1 -> Divide/1
  Math Function/1 -> Divide/2
  Vector Normal/1 -> Gain/1
  Cross Product/1 -> Gravity Gradient [N.m]/1
  Dot Product = magnitude squared/1 -> Math Function/1
  Gain/1 -> product 2/2
  product 2/1 -> Cross Product/2
  J/1 -> product 2/1
  Attitude (DCMi2b)/1 -> product 1/1
  product 1/1 -> Vector Normal/1, Gain1/1
  Gain1/1 -> Product (not cross)/1
  "Position (X) [m] "/1 -> product 1/2, Dot Product = magnitude squared/2, Dot Product = magnitude squared/1

== system Control_v6_LQR_2020b/Disturbance Torques/Magnetic Torque Model ==
  note: T = m X B
  note: B_earth [body]
  note: ECI to Body
  B (ECI) : Inport
  Attitude (DCMi2b) : Inport  Port=2
  Cross Product : vrlib/Utilities/Cross Product
  Product : Product  Multiplication=Matrix(*)  RndMeth=Zero
  constant : Constant  Value=sat.residual_dipole
  MagneticTorque (N.m) : Outport
  wires:
  Product/1 -> Cross Product/2
  Cross Product/1 -> MagneticTorque (N.m)/1
  constant/1 -> Cross Product/1
  Attitude (DCMi2b)/1 -> Product/1
  B (ECI)/1 -> Product/2

== system Control_v6_LQR_2020b/IGRF Computation block/Obtain B_ECI ==
  In1 : Inport
  Dipole Subsystem : Subsystem  TreatAsAtomicUnit=on
  IGRF Subsystem : Subsystem  TreatAsAtomicUnit=on
  If : If
  Merge : Merge
  Use_IGRF : Constant  Value=Use_IGRF
  u : Outport  VectorParamsAs1DForOutWhenUnconnected=off
  wires:
  If/1 -> IGRF Subsystem/Action
  In1/1 -> Dipole Subsystem/1(In1), IGRF Subsystem/1(In1)
  IGRF Subsystem/1(Out1) -> Merge/1
  Use_IGRF/1 -> If/1
  Merge/1 -> u/1
  Dipole Subsystem/1("B_ECI ") -> Merge/2
  If/2 -> Dipole Subsystem/Action

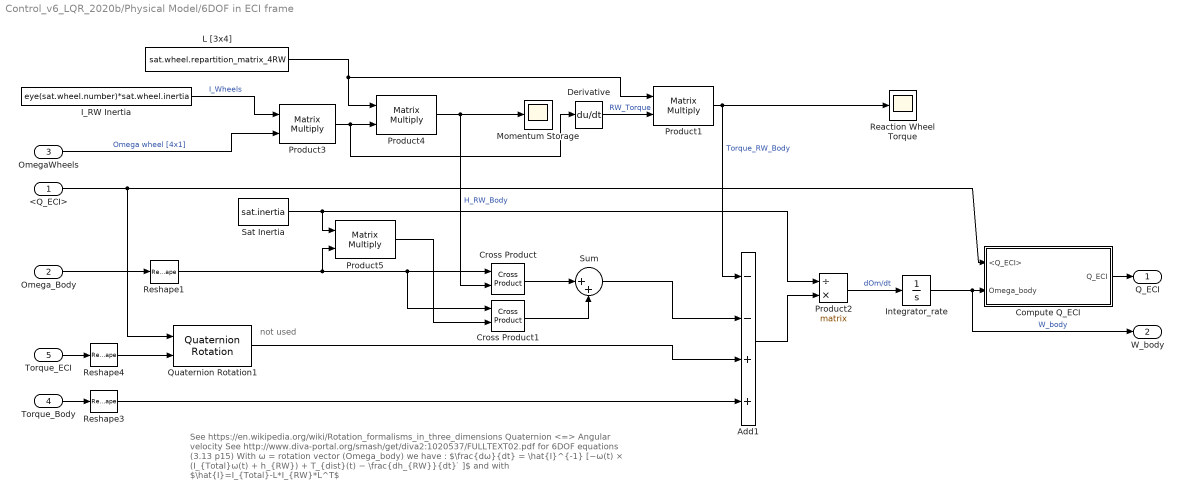
== system Control_v6_LQR_2020b/Physical Model/6DOF in ECI frame ==
  note: not used
  note: See https://en.wikipedia.org/wiki/Rotation_formalisms_in_three_dimensions Quaternion <=> Angular velocity
      |
      | See http://www.diva-portal.org/smash/get/diva2:1020537/FULLTEXT02.pdf for 6DOF equations (3.13 p15)
      |
      | With ω = rotation vector (Omega_body) we have :
      |
      | $\frac{dω}{dt} = \hat{I}^{-1} [−ω(t) × (I_{Total}ω(t) + h_{RW}) + T_{dist}(t) − \frac{dh_{RW}}{dt} ̇ ]$
      | and with $\hat{I}=I_{Total}-L*I_{RW}*L^T$
  <Q_ECI> : Inport
  "Omega_Body " : Inport  Port=2
  OmegaWheels : Inport  Port=3
  Torque_Body : Inport  Port=4
  Torque_ECI : Inport  Port=5  PortDimensions=3
  Add1 : Sum  Inputs=--++
  Compute Q_ECI : Subsystem
  Cross Product : vrlib/Utilities/Cross Product
  Cross Product1 : vrlib/Utilities/Cross Product
  Derivative : Derivative
  I_RW Inertia : Constant  Value=eye(sat.wheel.number)*sat.wheel.inertia
  Integrator_rate : Integrator
  L [3x4] : Constant  Value=sat.wheel.repartition_matrix_4RW
  Momentum Storage : Scope
  Product{1,3..5} (4 alike) : Product  Multiplication=Matrix(*)
  Product2 : Product  Inputs=/*  Multiplication=Matrix(*)
  Quaternion Rotation1 : aerolibutil/Quaternion Rotation
  Reaction Wheel Torque : Scope
  Reshape1 : Reshape  OutputDimensionality=Column vector (2-D)
  Reshape3 : Reshape  OutputDimensionality=Column vector (2-D)
  Reshape4 : Reshape  OutputDimensionality=Column vector (2-D)
  Sat Inertia : Constant  Value=sat.inertia
  Sum : Sum  Inputs=|++
  Q_ECI : Outport  VectorParamsAs1DForOutWhenUnconnected=off
  W_body : Outport  Port=2  VectorParamsAs1DForOutWhenUnconnected=off
  wires:
  Product2/1 -> Integrator_rate/1  "dOm/dt"
  Product3/1 -> Derivative/1, Product4/2
  Sat Inertia/1 -> Product5/1, Product2/1
  Add1/1 -> Product2/2
  Cross Product/1 -> Sum/1
  "Omega_Body "/1 -> Reshape1/1
  Integrator_rate/1 -> W_body/1, Compute Q_ECI/2(Omega_body)  "W_body"
  I_RW Inertia/1 -> Product3/1  "I_Wheels"
  Torque_Body/1 -> Reshape3/1
  Product1/1 -> Add1/1, Reaction Wheel Torque/1  "Torque_RW_Body"
  OmegaWheels/1 -> Product3/2  "Omega wheel [4x1]"
  Compute Q_ECI/1(Q_ECI) -> Q_ECI/1
  Torque_ECI/1 -> Reshape4/1
  <Q_ECI>/1 -> Quaternion Rotation1/1, Compute Q_ECI/1(<Q_ECI>)
  Quaternion Rotation1/1 -> Add1/3
  L [3x4]/1 -> Product1/1, Product4/1
  Reshape3/1 -> Add1/4
  Reshape4/1 -> Quaternion Rotation1/2
  Product4/1 -> Momentum Storage/1, Cross Product/2  "H_RW_Body"
  Reshape1/1 -> Product5/2, Cross Product1/1, Cross Product/1
  Derivative/1 -> Product1/2  "RW_Torque"
  Sum/1 -> Add1/2
  Cross Product1/1 -> Sum/2
  Product5/1 -> Cross Product1/2

== system Control_v6_LQR_2020b/Physical Model/Magnetorquer physics ==
  note: On pourrait aussi changer les blocs
      | magnétocoupleurs pour sortir les intensités
  Mag vector command : Inport
  B_IGRF_body (vecteur) : Inport  Port=2
  Add1 : Sum  Inputs=+++
  Cross Product : vrlib/Utilities/Cross Product
  Demux : Demux  Outputs=3
  Magnétocoupleur 1 : Subsystem
  Magnétocoupleur 2 : Subsystem
  Magnétocoupleur 3 : Subsystem
  Couple (vect) : Outport  PortDimensions=3  VectorParamsAs1DForOutWhenUnconnected=off
  Real mag moments vector : Outport  Port=2  VectorParamsAs1DForOutWhenUnconnected=off
  wires:
  Add1/1 -> Real mag moments vector/1, Cross Product/1  "M_real"
  Demux/1 -> Magnétocoupleur 1/1(m_in (scalar))
  Demux/2 -> Magnétocoupleur 2/1(m_in (scalar))
  Demux/3 -> Magnétocoupleur 3/1(m_in (scalar))
  Mag vector command/1 -> Demux/1
  Magnétocoupleur 2/1(m_out (vect)) -> Add1/2
  Magnétocoupleur 1/1(m_out (vect)) -> Add1/1
  Magnétocoupleur 3/1(m_out (vect)) -> Add1/3
  Cross Product/1 -> Couple (vect)/1  "T_body"
  B_IGRF_body (vecteur)/1 -> Cross Product/2

== system Control_v6_LQR_2020b/Physical Model/Thruster ==
  On/Off (Boolean) : Inport  OutDataTypeStr=boolean
  Constant : Constant  Value=0
  Cross Product : vrlib/Utilities/Cross Product
  If : If  IfExpression=u1
  If Action Subsystem : Subsystem  TreatAsAtomicUnit=on
  If Action Subsystem1 : Subsystem  TreatAsAtomicUnit=on
  Merge : Merge
  Product : Product
  Sum : Sum  Inputs=|-+
  Thruster Force : Constant  Value=sat.thruster.force
  unit vector of thrust : Constant  Value=sat.thruster.dir
  vector CoG : Constant  Value=sat.CoG
  vector G-Thrust point : Constant  Value=sat.thruster.point
  Force (G_sat) : Outport  VectorParamsAs1DForOutWhenUnconnected=off
  Moment (G_sat) : Outport  Port=2  VectorParamsAs1DForOutWhenUnconnected=off
  wires:
  Product/1 -> Force (G_sat)/1, Cross Product/2
  Sum/1 -> Cross Product/1
  unit vector of thrust/1 -> Product/1
  Cross Product/1 -> Moment (G_sat)/1
  Thruster Force/1 -> If Action Subsystem/1(In1)
  On/Off (Boolean)/1 -> If/1
  If/1 -> If Action Subsystem/Action
  If/2 -> If Action Subsystem1/Action
  If Action Subsystem1/1(Out1) -> Merge/2
  If Action Subsystem/1(Out1) -> Merge/1
  Merge/1 -> Product/2
  Constant/1 -> If Action Subsystem1/1(In1)
  vector G-Thrust point/1 -> Sum/1
  vector CoG/1 -> Sum/2

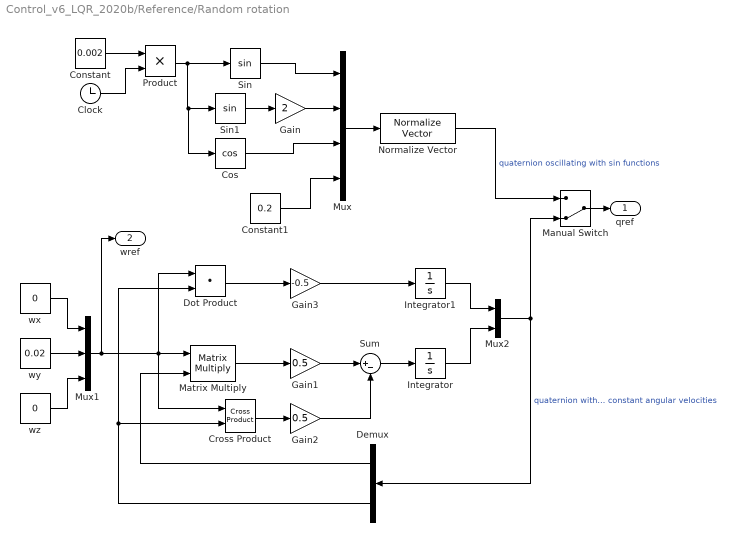
== system Control_v6_LQR_2020b/Reference/Random rotation ==
  Clock : Clock
      settings: Decimation=TimeStep
  Constant : Constant  Value=0.002
  Constant1 : Constant  Value=0.2
  Cos : Trigonometry  Operator=cos
  Cross Product : vrlib/Utilities/Cross Product
  Demux : Demux  Outputs=[1;3]
  Dot Product : DotProduct  InputSameDT=on  OutDataTypeStr=Inherit: Inherit via internal rule
  Gain : Gain  Gain=2
  Gain1 : Gain  Gain=0.5
  Gain2 : Gain  Gain=0.5
  Gain3 : Gain  Gain=-0.5
  Integrator : Integrator  InitialCondition=[0;0;0]
  Integrator1 : Integrator  InitialCondition=1
  Manual Switch : ManualSwitch  CurrentSetting=0
  Matrix Multiply : Product  Multiplication=Matrix(*)
  Mux : Mux
  Mux1 : Mux  Inputs=3
  Mux2 : Mux  Inputs=[1;3]
  Normalize Vector : vrlib/Utilities/Normalize Vector  maxzero=0
  Product : Product
  Sin : Trigonometry
  Sin1 : Trigonometry
  Sum : Sum  Inputs=|+-
  wx : Constant  Value=0
  wy : Constant  Value=0.02
  wz : Constant  Value=0
  qref : Outport
  wref : Outport  Port=2
  wires:
  Mux/1 -> Normalize Vector/1
  Normalize Vector/1 -> Manual Switch/1  "quaternion oscillating with sin functions"
  Constant/1 -> Product/1
  Clock/1 -> Product/2
  Product/1 -> Cos/1, Sin1/1, Sin/1
  Sin/1 -> Mux/1
  Sin1/1 -> Gain/1
  Gain/1 -> Mux/2
  Cos/1 -> Mux/3
  Constant1/1 -> Mux/4
  Manual Switch/1 -> qref/1
  wx/1 -> Mux1/1
  wy/1 -> Mux1/2
  wz/1 -> Mux1/3
  Mux1/1 -> wref/1, Dot Product/1, Cross Product/1, Matrix Multiply/1
  Matrix Multiply/1 -> Gain1/1
  Gain1/1 -> Sum/1
  Sum/1 -> Integrator/1
  Integrator/1 -> Mux2/2
  Mux2/1 -> Demux/1, Manual Switch/2  "quaternion with constant angular velocities"
  Demux/1 -> Matrix Multiply/2
  Cross Product/1 -> Gain2/1
  Gain2/1 -> Sum/2
  Dot Product/1 -> Gain3/1
  Gain3/1 -> Integrator1/1
  Integrator1/1 -> Mux2/1
  Demux/2 -> Cross Product/2, Dot Product/2

== system Control_v6_LQR_2020b/Reference/Switch Case Action Subsystem ==
  Q_orbit : Inport
  W_orbit1 : Inport  Port=2
  Action Port : ActionPort  ActionPortLabel=default:
  Out1 : Outport  VectorParamsAs1DForOutWhenUnconnected=off
  Out3 : Outport  Port=2  VectorParamsAs1DForOutWhenUnconnected=off
  wires:
  Q_orbit/1 -> Out1/1
  W_orbit1/1 -> Out3/1

== system Control_v6_LQR_2020b/Reference/Switch Case Action Subsystem1 ==
  Q_retro : Inport
  W_retro : Inport  Port=2
  Action Port : ActionPort  ActionPortLabel=case [ 5 ]:
  Out1 : Outport  VectorParamsAs1DForOutWhenUnconnected=off
  Out3 : Outport  Port=2  VectorParamsAs1DForOutWhenUnconnected=off
  wires:
  Q_retro/1 -> Out1/1
  W_retro/1 -> Out3/1

== system Control_v6_LQR_2020b/Reference/Switch Case Action Subsystem2 ==
  note: q from I to O + rotation
  Q_drag : Inport
  W_drag : Inport  Port=2
  Action Port : ActionPort  ActionPortLabel=case [ 4 ]:
  Out1 : Outport  VectorParamsAs1DForOutWhenUnconnected=off
  W : Outport  Port=2
  wires:
  Q_drag/1 -> Out1/1
  W_drag/1 -> W/1

== system Control_v6_LQR_2020b/Reference/Switch Case Action Subsystem3 ==
  Q_sun_sun : Inport
  W_sun_sun : Inport  Port=2
  Action Port : ActionPort  ActionPortLabel=case [ 3 ]:
  Out1 : Outport  VectorParamsAs1DForOutWhenUnconnected=off
  Out3 : Outport  Port=2  VectorParamsAs1DForOutWhenUnconnected=off
  wires:
  Q_sun_sun/1 -> Out1/1
  W_sun_sun/1 -> Out3/1

== system Control_v6_LQR_2020b/Reference/Switch Case Action Subsystem4 ==
  Q_sun_aero : Inport
  W_sun_aero : Inport  Port=2
  Action Port : ActionPort  ActionPortLabel=case [ 2 ]:
  Out1 : Outport  VectorParamsAs1DForOutWhenUnconnected=off
  Out3 : Outport  Port=2  VectorParamsAs1DForOutWhenUnconnected=off
  wires:
  Q_sun_aero/1 -> Out1/1
  W_sun_aero/1 -> Out3/1

== system Control_v6_LQR_2020b/Reference/Switch Case Action Subsystem5 ==
  In1 : Inport
  W_orbit : Inport  Port=2
  Action Port : ActionPort  ActionPortLabel=case [ 1 ]:
  Out1 : Outport  VectorParamsAs1DForOutWhenUnconnected=off
  Out3 : Outport  Port=2  VectorParamsAs1DForOutWhenUnconnected=off
  wires:
  In1/1 -> Out1/1
  W_orbit/1 -> Out3/1

== system Control_v6_LQR_2020b/Reference/Switch Case Action Subsystem6 ==
  In1 : Inport
  In2 : Inport  Port=2
  Action Port : ActionPort  ActionPortLabel=case [ 7 ]:
  Derivative : Derivative
  Matrix Multiply : Product  Multiplication=Matrix(*)
  Quaternions to Direction Cosine Matrix : sharedtransform/Quaternions to  Direction Cosine Matrix  aMode=aMode
      settings: SourceProductBaseCode=AE,PW,DR,MT,UV,VE
  Transpose : Math  Operator=transpose  SaturateOnIntegerOverflow=on
  Transpose1 : Math  Operator=transpose  SaturateOnIntegerOverflow=on
  gets vector from Skew Matrix : MATLABFcn  MATLABFcn=vec_from_skew
  Out1 : Outport  VectorParamsAs1DForOutWhenUnconnected=off
  W_custom : Outport  Port=2
  wires:
  In1/1 -> Out1/1
  In2/1 -> Quaternions to Direction Cosine Matrix/1
  Quaternions to Direction Cosine Matrix/1 -> Transpose1/1
  Matrix Multiply/1 -> gets vector from Skew Matrix/1
  Transpose/1 -> Derivative/1
  gets vector from Skew Matrix/1 -> W_custom/1
  Derivative/1 -> Matrix Multiply/1
  Transpose1/1 -> Transpose/1, Matrix Multiply/2

== system Control_v6_LQR_2020b/Reference/Switch Case Action Subsystem7 ==
  In1 : Inport
  In2 : Inport  Port=2
  Action Port : ActionPort  ActionPortLabel=case [ 6 ]:
  Out1 : Outport  VectorParamsAs1DForOutWhenUnconnected=off
  Out2 : Outport  Port=2  VectorParamsAs1DForOutWhenUnconnected=off
  wires:
  In1/1 -> Out1/1
  In2/1 -> Out2/1

== system Control_v6_LQR_2020b/Reference/Switch Case Action Subsystem8 ==
  Q_retro : Inport
  W_retro : Inport  Port=2
  Action Port : ActionPort  ActionPortLabel=case [ 8 ]:
  Out1 : Outport  VectorParamsAs1DForOutWhenUnconnected=off
  Out3 : Outport  Port=2  VectorParamsAs1DForOutWhenUnconnected=off
  wires:
  Q_retro/1 -> Out1/1
  W_retro/1 -> Out3/1

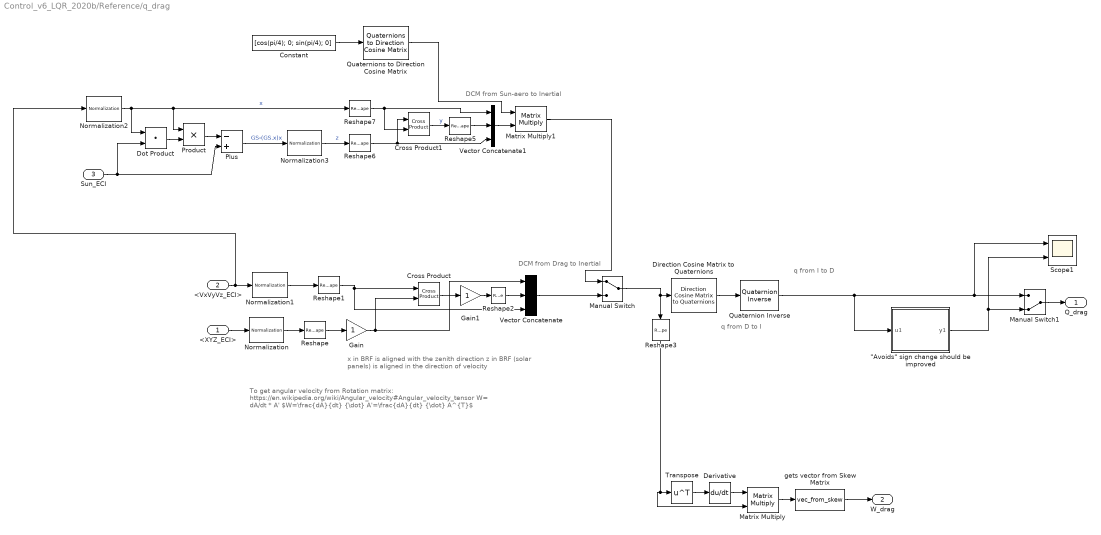
== system Control_v6_LQR_2020b/Reference/q_drag ==
  note: x in BRF is aligned with the zenith direction
      | z in BRF (solar panels) is aligned in the direction of velocity
  note: DCM from Drag to Inertial
  note: q from D to I
  note: q from I to D
  note: To get angular velocity from Rotation matrix:
      | https://en.wikipedia.org/wiki/Angular_velocity#Angular_velocity_tensor
      | W= dA/dt * A'
      | $W=\frac{dA}{dt} {\dot} A'=\frac{dA}{dt} {\dot} A^{T}$
  note: DCM from Sun-aero to Inertial
  <XYZ_ECI> : Inport
  <VxVyVz_ECI> : Inport  Port=2
  Sun_ECI : Inport  Port=3
  "\"Avoids\" sign change should be improved" : Subsystem
  Constant : Constant  Value=[cos(pi/4); 0; sin(pi/4); 0]
  Cross Product : vrlib/Utilities/Cross Product
  Cross Product1 : vrlib/Utilities/Cross Product
  Derivative : Derivative
  Direction Cosine Matrix to Quaternions : sharedtransform/Direction Cosine Matrix  to Quaternions  aMode=0  action=None  tolerance=eps(2)
      settings: SourceProductBaseCode=AE,PW,DR,MT,UV,VE
  Dot Product : DotProduct  InputSameDT=on  OutDataTypeStr=Inherit: Inherit via internal rule
  Gain : Gain
  Gain1 : Gain
  Manual Switch : ManualSwitch
  Manual Switch1 : ManualSwitch  CurrentSetting=0
  Matrix Multiply : Product  Multiplication=Matrix(*)
  Matrix Multiply1 : Product  Multiplication=Matrix(*)
  Normalization{,1..3} (4 alike) : dspmathops/Normalization  NormType=2-norm  Bias=1e-10  NormOver=Each column  Dimension=1  roundingMode=Floor  overflowMode=off  accumDataTypeStr=Inherit: Same as product output  accumLastDataTypeStr=Inherit: Same as product output  outputDataTypeStr=Inherit: Same as product output  outputMin=[]  outputMax=[]  outputLastDataTypeStr=Inherit: Same as product output
  Plus : Sum  Inputs=-+
  Product : Product
  Quaternion Inverse : aerolibutil/Quaternion Inverse
  Quaternions to Direction Cosine Matrix : sharedtransform/Quaternions to  Direction Cosine Matrix  aMode=aMode
      settings: SourceProductBaseCode=AE,PW,DR,MT,UV,VE
  Reshape{,1..2,5..7} (6 alike) : Reshape  OutputDimensionality=Column vector (2-D)
  Reshape3 : Reshape  OutputDimensionality=Customize  OutputDimensions=[3,3]
  Scope1 : Scope  NumInputPorts=2
  Transpose : Math  Operator=transpose  SaturateOnIntegerOverflow=on
  Vector Concatenate : Concatenate  NumInputs=3  Mode=Multidimensional array  ConcatenateDimension=2
  Vector Concatenate1 : Concatenate  NumInputs=3  Mode=Multidimensional array  ConcatenateDimension=2
  gets vector from Skew Matrix : MATLABFcn  MATLABFcn=vec_from_skew
  Q_drag : Outport  VectorParamsAs1DForOutWhenUnconnected=off
  W_drag : Outport  Port=2
  wires:
  Normalization/1 -> Reshape/1
  Normalization1/1 -> Reshape1/1
  Reshape1/1 -> Cross Product/1, Vector Concatenate/3
  <XYZ_ECI>/1 -> Normalization/1
  Reshape/1 -> Gain/1
  Gain/1 -> Cross Product/2, Vector Concatenate/1
  Direction Cosine Matrix to Quaternions/1 -> Quaternion Inverse/1
  Cross Product/1 -> Gain1/1
  Gain1/1 -> Reshape2/1
  Quaternion Inverse/1 -> "\"Avoids\" sign change should be improved"/1(u1), Manual Switch1/1, Scope1/1
  Manual Switch/1 -> Reshape3/1, Direction Cosine Matrix to Quaternions/1
  gets vector from Skew Matrix/1 -> W_drag/1
  Matrix Multiply/1 -> gets vector from Skew Matrix/1
  Transpose/1 -> Derivative/1
  Derivative/1 -> Matrix Multiply/1
  Reshape2/1 -> Vector Concatenate/2
  Reshape3/1 -> Matrix Multiply/2, Transpose/1
  "\"Avoids\" sign change should be improved"/1(y1) -> Manual Switch1/2, Scope1/2
  Manual Switch1/1 -> Q_drag/1
  Reshape6/1 -> Vector Concatenate1/3, Cross Product1/1
  Product/1 -> Plus/1
  Cross Product1/1 -> Reshape5/1  "y"
  Sun_ECI/1 -> Dot Product/2, Plus/2
  Dot Product/1 -> Product/2
  Reshape5/1 -> Vector Concatenate1/2
  Reshape7/1 -> Vector Concatenate1/1, Cross Product1/2
  Normalization3/1 -> Reshape6/1  "z"
  Normalization2/1 -> Dot Product/1, Product/1, Reshape7/1  "x"
  Plus/1 -> Normalization3/1  "GS-(GS.x)x"
  Vector Concatenate1/1 -> Matrix Multiply1/2
  Quaternions to Direction Cosine Matrix/1 -> Matrix Multiply1/1
  Constant/1 -> Quaternions to Direction Cosine Matrix/1
  Matrix Multiply1/1 -> Manual Switch/1
  <VxVyVz_ECI>/1 -> Normalization2/1, Normalization1/1
  Vector Concatenate/1 -> Manual Switch/2
